simulink model "Mounna_CollecteurAdm"  (R2024b)
settings: Solver=VariableStepAuto  StartTime=0.0  StopTime=10.0  RelTol=1e-3
undefined symbols (not defined in the file): DebitAirEvt, DebitMoteurEvt, ManifoldMassTest, ManifoldPressureTest, ManifoldTemperatureTest, ManifoldTimeTest, Rair, Tamb, TempsEvt, Vcol
settings Model: Creator=a030141  LastModifiedBy=ramse
settings DebuggingCC: UnderspecifiedInitializationDetection=Classic  MergeDetectMultiDrivingBlocksExec=none
settings ModelReferenceCC: PropagateSignalLabelsOutOfModel=off

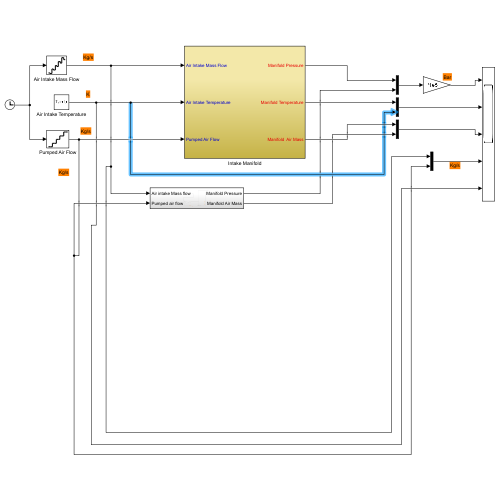
[thumbnail: Simulink's stored preview of the top-level diagram]
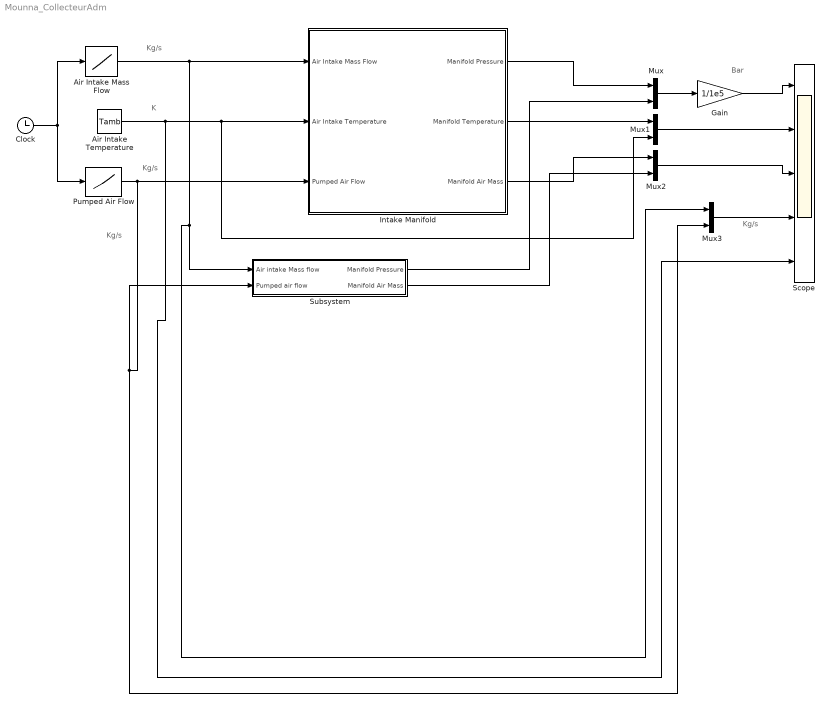
== system Mounna_CollecteurAdm ==
  note: Kg/s
  note: Kg/s
  note: Kg/s
  note: K
  note: Bar
  note: Kg/s
  Air Intake Mass Flow : Lookup  InputValues=TempsEvt  Table=DebitAirEvt
  Air Intake Temperature : Constant  Value=Tamb
  Clock : Clock
  Gain : Gain  Gain=1/1e5  SaturateOnIntegerOverflow=on  OutDataTypeStr=Inherit: Same as input  ParamDataTypeStr=Inherit: Same as input
  Intake Manifold : Subsystem
  Mux{,1..3} (4 alike) : Mux  Inputs=2
  Pumped Air Flow : Lookup  InputValues=TempsEvt  Table=DebitMoteurEvt
  Scope : Scope  NumInputPorts=5
  Subsystem : Subsystem
  wires:
  Air Intake Temperature/1 -> Scope/5, Mux1/2, Intake Manifold/2(Air Intake Temperature)
  Clock/1 -> Pumped Air Flow/1, Air Intake Mass Flow/1
  Air Intake Mass Flow/1 -> Subsystem/1(Air intake Mass flow), Mux3/1, Intake Manifold/1(Air Intake Mass Flow)
  Pumped Air Flow/1 -> Mux3/2, Subsystem/2(Pumped air flow), Intake Manifold/3(Pumped Air Flow)
  Mux/1 -> Gain/1
  Gain/1 -> Scope/1
  Mux1/1 -> Scope/2
  Mux2/1 -> Scope/3
  Mux3/1 -> Scope/4
  Intake Manifold/1(Manifold Pressure) -> Mux/1
  Intake Manifold/2(Manifold Temperature) -> Mux1/1
  Intake Manifold/3(Manifold Air Mass) -> Mux2/1
  Subsystem/1(Manifold Pressure) -> Mux/2
  Subsystem/2(Manifold Air Mass) -> Mux2/2

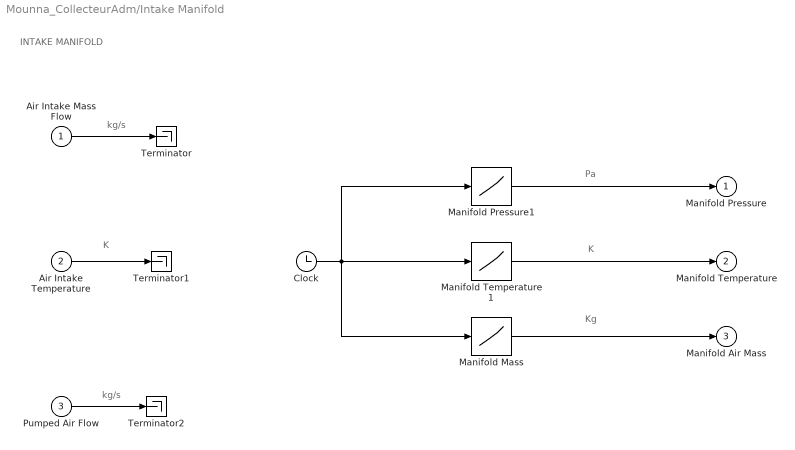
== system Mounna_CollecteurAdm/Intake Manifold ==
  note: INTAKE MANIFOLD
  note: kg/s
  note: K
  note: kg/s
  note: Kg
  note: K
  note: Pa
  Air Intake Mass Flow : Inport
  Air Intake Temperature : Inport  Port=2
  Pumped Air Flow : Inport  Port=3
  Clock : Clock
  Manifold Mass : Lookup  InputValues=ManifoldTimeTest  Table=ManifoldMassTest
  Manifold Pressure1 : Lookup  InputValues=ManifoldTimeTest  Table=ManifoldPressureTest
  Manifold Temperature1 : Lookup  InputValues=ManifoldTimeTest  Table=ManifoldTemperatureTest
  Terminator : Terminator
  Terminator1 : Terminator
  Terminator2 : Terminator
  Manifold Pressure : Outport
  Manifold Temperature : Outport  Port=2
  Manifold Air Mass : Outport  Port=3
  wires:
  Pumped Air Flow/1 -> Terminator2/1
  Air Intake Mass Flow/1 -> Terminator/1
  Air Intake Temperature/1 -> Terminator1/1
  Manifold Pressure1/1 -> Manifold Pressure/1
  Manifold Temperature1/1 -> Manifold Temperature/1
  Manifold Mass/1 -> Manifold Air Mass/1
  Clock/1 -> Manifold Temperature1/1, Manifold Pressure1/1, Manifold Mass/1

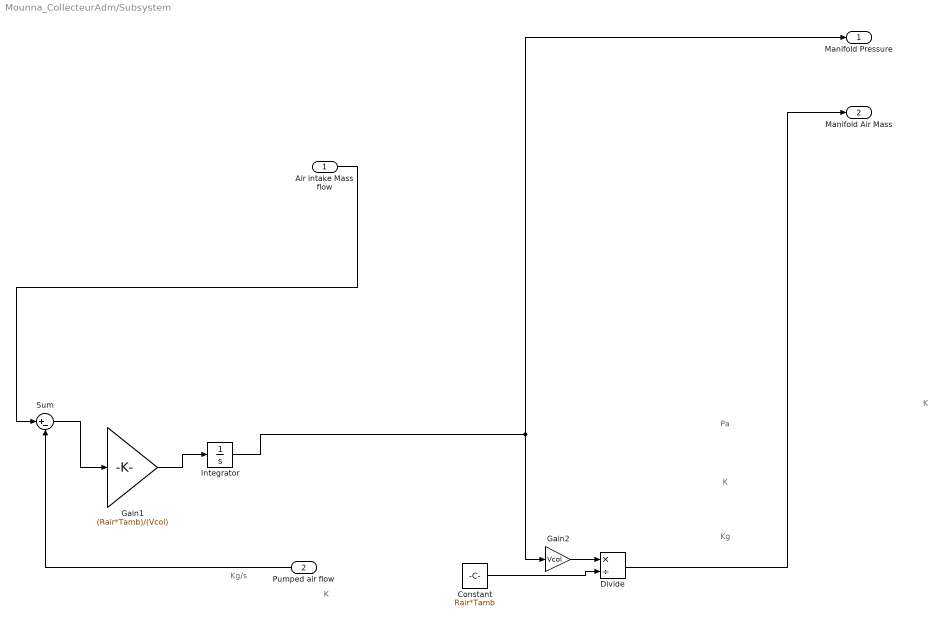
== system Mounna_CollecteurAdm/Subsystem ==
  note: Kg/s
  note: Kg
  note: K
  note: Pa
  note: K
  note: K
  Air intake Mass flow : Inport
  Pumped air flow : Inport  Port=2
  Constant : Constant  Value=Rair*Tamb
  Divide : Product  Inputs=*/
  Gain1 : Gain  Gain=(Rair*Tamb)/(Vcol)
  Gain2 : Gain  Gain=Vcol
  Integrator : Integrator
  Sum : Sum  Inputs=|+-
  Manifold Pressure : Outport
  Manifold Air Mass : Outport  Port=2
  wires:
  Gain2/1 -> Divide/1
  Air intake Mass flow/1 -> Sum/1
  Sum/1 -> Gain1/1
  Divide/1 -> Manifold Air Mass/1
  Gain1/1 -> Integrator/1
  Pumped air flow/1 -> Sum/2
  Constant/1 -> Divide/2
  Integrator/1 -> Manifold Pressure/1, Gain2/1
